simulink model "Mapa_Discreto"  (R2017a)
settings: Solver=VariableStepAuto  StartTime=0.0  StopTime=10.0  RelTol=1e-3
undefined symbols (not defined in the file or in its folder): a11, a12, a21, a22
libraries: simulink x1
settings Model: Creator=franj  LastModifiedBy=franj

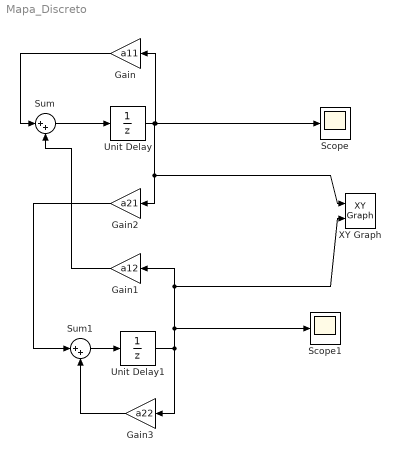
== system Mapa_Discreto ==
  Gain : Gain  Gain=a11
  Gain1 : Gain  Gain=a12
  Gain2 : Gain  Gain=a21
  Gain3 : Gain  Gain=a22
  Scope : Scope
  Scope1 : Scope
  Sum : Sum  Inputs=|++
  Sum1 : Sum  Inputs=|++
  Unit Delay : UnitDelay  InitialCondition=1  SampleTime=-1
  Unit Delay1 : UnitDelay  InitialCondition=1  SampleTime=-1
  XY Graph : simulink/Sinks/XY Graph  xmin=-1  xmax=1  ymin=-1  ymax=1  st=-1
  wires:
  Sum/1 -> Unit Delay/1
  Unit Delay/1 -> Scope/1, Gain/1, XY Graph/1, Gain2/1
  Unit Delay1/1 -> XY Graph/2, Gain1/1, Scope1/1, Gain3/1
  Gain1/1 -> Sum/2
  Gain/1 -> Sum/1
  Sum1/1 -> Unit Delay1/1
  Gain2/1 -> Sum1/1
  Gain3/1 -> Sum1/2
